simulink model "samp"  (R2013a)
settings: Solver=FixedStepDiscrete  StartTime=0.0  StopTime=10.0  FixedStep=Ts  RelTol=1e-3
values from neighbouring files (symbols this model uses):
  seed = rand(1)    [discrete_markov_system_response_h2_rob_poly_control_input.m]
  Ts = t(2)-t(1)    [discrete_markov_system_response_h2_rob.m]    (also in discrete_markov_system_response_h2_rob_poly_control_input.m = 0.05; discrete_markov_system_response_hinf_rob.m; main_h2_rob.m = 0.05)
libraries: simulink x2
settings Model: Creator=amarc  LastModifiedBy=amarc
settings DataIOCC: LimitDataPoints=off

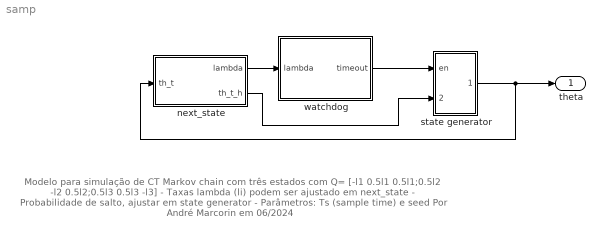
== system samp ==
  note: Modelo para simulação de CT Markov chain com três estados
      | com Q= [-l1 0.5l1 0.5l1;0.5l2 -l2 0.5l2;0.5l3 0.5l3 -l3]
      | - Taxas lambda (li) podem ser ajustado em next_state
      | - Probabilidade de salto, ajustar em state generator
      | - Parâmetros: Ts (sample time) e seed
      | Por André Marcorin em 06/2024
  "next_state " : Subsystem
  state generator : Subsystem
  watchdog : Subsystem
  theta : Outport
  wires:
  "next_state "/1(lambda) -> watchdog/1(lambda)
  watchdog/1(timeout) -> state generator/1(en)
  "next_state "/2(th_t_h) -> state generator/2(next)
  state generator/1(theta) -> "next_state "/1(th_t), theta/1

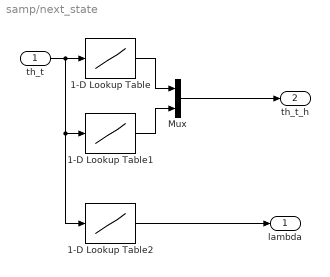
== system samp/next_state  ==
  th_t : Inport
  1-D Lookup Table : Lookup_n-D  NumberOfTableDimensions=1  BreakpointsForDimension1=[1:3]  Table=[2 1 3]  RndMeth=Simplest  InputSameDT=on
  1-D Lookup Table1 : Lookup_n-D  NumberOfTableDimensions=1  BreakpointsForDimension1=[1:3]  Table=[3 3 2]  RndMeth=Simplest  InputSameDT=on
  1-D Lookup Table2 : Lookup_n-D  NumberOfTableDimensions=1  BreakpointsForDimension1=[1:3]  Table=[1 2 4]  RndMeth=Simplest  InputSameDT=on
  Mux : Mux  Inputs=2
  lambda : Outport
  th_t_h : Outport  Port=2
  wires:
  1-D Lookup Table1/1 -> Mux/2
  1-D Lookup Table/1 -> Mux/1
  Mux/1 -> th_t_h/1
  th_t/1 -> 1-D Lookup Table2/1, 1-D Lookup Table1/1, 1-D Lookup Table/1
  1-D Lookup Table2/1 -> lambda/1

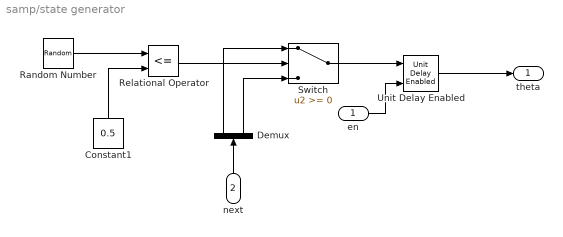
== system samp/state generator ==
  en : Inport
  next : Inport  Port=2
  Constant1 : Constant  Value=0.5
  Demux : Demux  Outputs=2
  Random Number : RandomNumber  SampleTime=Ts
  Relational Operator : RelationalOperator  Operator=<=  OutDataTypeStr=boolean
  Switch : Switch
  Unit Delay Enabled : simulink/Additional Math & Discrete/Additional Discrete/Unit Delay Enabled  vinit=1  tsamp=-1
  theta : Outport
  wires:
  Random Number/1 -> Relational Operator/1
  Constant1/1 -> Relational Operator/2
  Relational Operator/1 -> Switch/2
  en/1 -> Unit Delay Enabled/2
  Unit Delay Enabled/1 -> theta/1
  Switch/1 -> Unit Delay Enabled/1
  Demux/1 -> Switch/1
  Demux/2 -> Switch/3
  next/1 -> Demux/1

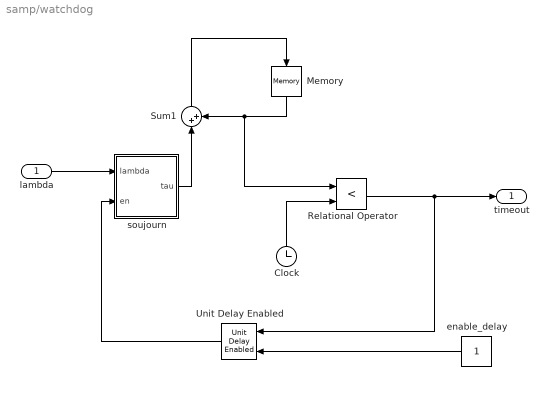
== system samp/watchdog ==
  lambda : Inport
  Clock : Clock
  Memory : Memory
  Relational Operator : RelationalOperator  Operator=<  OutDataTypeStr=boolean
  Sum1 : Sum  Inputs=|++
  Unit Delay Enabled : simulink/Additional Math & Discrete/Additional Discrete/Unit Delay Enabled  vinit=1  tsamp=-1
  enable_delay : Constant
  soujourn : Subsystem
  timeout : Outport
  wires:
  enable_delay/1 -> Unit Delay Enabled/2
  Sum1/1 -> Memory/1
  Memory/1 -> Relational Operator/1, Sum1/2
  soujourn/1(tau) -> Sum1/1
  lambda/1 -> soujourn/1(lambda)
  Clock/1 -> Relational Operator/2
  Relational Operator/1 -> timeout/1, Unit Delay Enabled/1
  Unit Delay Enabled/1 -> soujourn/2(en)

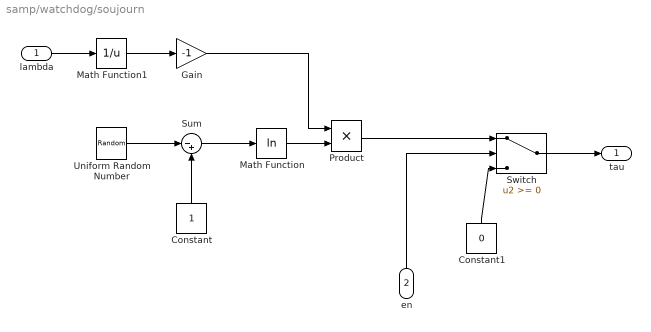
== system samp/watchdog/soujourn ==
  lambda : Inport
  en : Inport  Port=2
  Constant : Constant
  Constant1 : Constant  Value=0
  Gain : Gain  Gain=-1
  Math Function : Math  Operator=log  SaturateOnIntegerOverflow=on
  Math Function1 : Math  Operator=reciprocal  SaturateOnIntegerOverflow=on
  Product : Product
  Sum : Sum  Inputs=|-+
  Switch : Switch
  Uniform Random Number : UniformRandomNumber  Minimum=0  Seed=seed  SampleTime=Ts
  tau : Outport
  wires:
  Uniform Random Number/1 -> Sum/1
  Constant/1 -> Sum/2
  Math Function1/1 -> Gain/1
  lambda/1 -> Math Function1/1
  en/1 -> Switch/2
  Sum/1 -> Math Function/1
  Gain/1 -> Product/1
  Math Function/1 -> Product/2
  Product/1 -> Switch/1
  Constant1/1 -> Switch/3
  Switch/1 -> tau/1
